simulink model "freq_response_with_sweep"  (R2014b)
settings: Solver=FixedStepDiscrete  StartTime=0.0  StopTime=15  RelTol=1e-3
InitFcn:
  | fs=8000;
  | Ts=1/fs;
StopFcn:
  | tf_estimation
libraries: dspsrcs4 x2, dspindex x1, dspsnks4 x1
settings Model: Creator=wleonsal  LastModifiedBy=fritz2

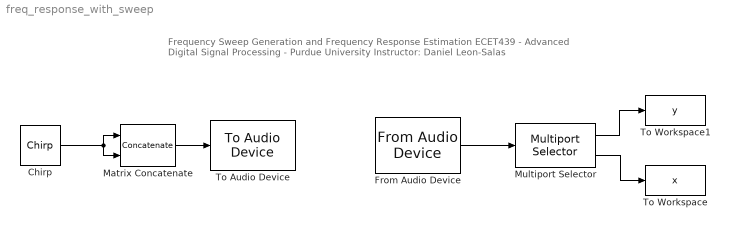
== system freq_response_with_sweep ==
  note: Frequency Sweep Generation and Frequency Response Estimation
      | ECET439 - Advanced Digital Signal Processing - Purdue University
      | Instructor: Daniel Leon-Salas
  Chirp : dspsrcs4/Chirp  sweep=Linear  mode=Unidirectional  f0=50  f1=fs/2  t1=10  Tsweep=10  phase=0  Ts=Ts  spf=1024  datatype=Double
  From Audio Device : dspsrcs4/From Audio Device  deviceName=Microphone (Realtek High Definition Audio)  numChannels=2  sampleRate=fs  deviceDatatype=Determine from output data type  autoBufferSize=on  bufferSize=4096  queueDuration=1.0  frameSize=1024  outputDatatype=double  defaultInputChannelMapping=on  inputChannelMapping=1:2  outputNumOverrunSamples=off
  Matrix Concatenate : Concatenate  Mode=Multidimensional array  ConcatenateDimension=2
  Multiport Selector : dspindex/Multiport Selector  rowsOrCols=Columns  idxCellArray={ 1, 2 }  idxErrMode=Clip Index
  To Audio Device : dspsnks4/To Audio Device  deviceName=Speakers / Headphones (Realtek High Definition Audio)  inheritSampleRate=on  sampleRate=44100  deviceDatatype=Determine from input data type  autoBufferSize=on  bufferSize=4096  queueDuration=1.0  defaultOutputChannelMapping=on  outputChannelMapping=1:2  outputNumUnderrunSamples=off
  To Workspace : ToWorkspace  VariableName=x  SaveFormat=Timeseries  SampleTime=-1
  To Workspace1 : ToWorkspace  VariableName=y  SaveFormat=Timeseries  SampleTime=-1
  wires:
  Matrix Concatenate/1 -> To Audio Device/1
  Chirp/1 -> Matrix Concatenate/2, Matrix Concatenate/1
  From Audio Device/1 -> Multiport Selector/1
  Multiport Selector/1 -> To Workspace1/1
  Multiport Selector/2 -> To Workspace/1
